simulink subsystem "button_filter"  (R2022b)
settings: Solver=VariableStepAuto  StartTime=0.0  StopTime=0.02  RelTol=1e-3
libraries: simulink x8
settings Model: DefaultTestHarness=button_filter_harness  Creator=andre  LastModifiedBy=andre
settings ModelReferenceCC: EnableRefExpFcnMdlSchedulingChecks=on

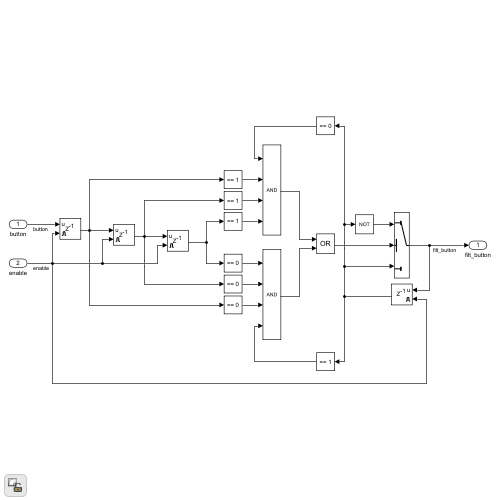
[thumbnail: Simulink's stored preview of the top-level diagram]
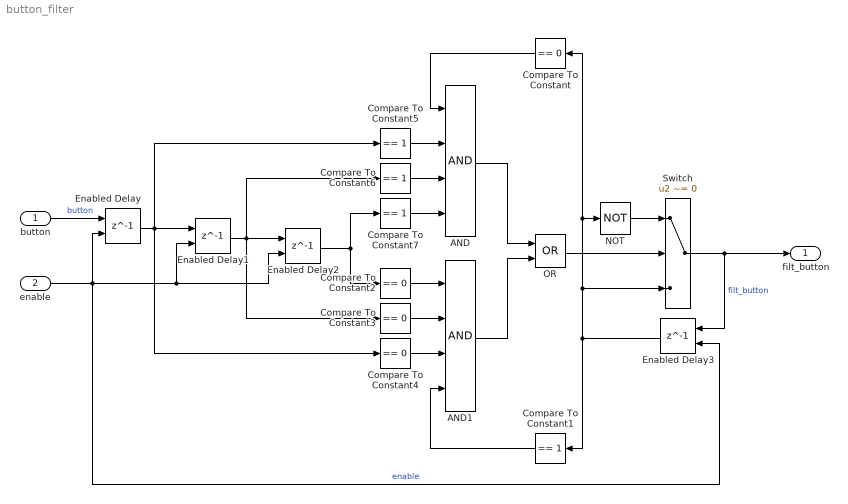
== system button_filter ==
  button : Inport  OutDataTypeStr=boolean  PortDimensions=1
  enable : Inport  Port=2  OutDataTypeStr=boolean  PortDimensions=1
  AND : Logic  Inputs=4  AllPortsSameDT=off  OutDataTypeStr=boolean
  AND1 : Logic  Inputs=4  AllPortsSameDT=off  OutDataTypeStr=boolean
  Compare To Constant{,2..4} (4 alike) : simulink/Logic and Bit Operations/Compare To Constant  relop===  const=0  OutDataTypeStr=boolean
  Compare To Constant{1,5..7} (4 alike) : simulink/Logic and Bit Operations/Compare To Constant  relop===  const=1  OutDataTypeStr=boolean
  Enabled Delay{,1..3} (4 alike) : Delay  DelayLength=1  ShowEnablePort=on
      settings: InputPortMap=u0,e6
  NOT : Logic  Operator=NOT  AllPortsSameDT=off  OutDataTypeStr=boolean
  OR : Logic  Operator=OR  AllPortsSameDT=off  OutDataTypeStr=boolean
  Switch : Switch  Criteria=u2 ~= 0  SaturateOnIntegerOverflow=off  InputSameDT=off
  filt_button : Outport  OutDataTypeStr=boolean  PortDimensions=1
  wires:
  button/1 -> Enabled Delay/1  "button"
  Switch/1 -> filt_button/1, Enabled Delay3/1  "filt_button"
  Compare To Constant3/1 -> AND1/2
  Compare To Constant1/1 -> AND1/4
  Enabled Delay2/1 -> Compare To Constant2/1, Compare To Constant7/1
  Enabled Delay3/1 -> Switch/3, NOT/1, Compare To Constant/1, Compare To Constant1/1
  AND1/1 -> OR/2
  Compare To Constant6/1 -> AND/3
  Compare To Constant7/1 -> AND/4
  OR/1 -> Switch/2
  Compare To Constant/1 -> AND/1
  AND/1 -> OR/1
  Enabled Delay/1 -> Compare To Constant5/1, Enabled Delay1/1, Compare To Constant4/1
  Compare To Constant4/1 -> AND1/3
  Compare To Constant2/1 -> AND1/1
  Compare To Constant5/1 -> AND/2
  NOT/1 -> Switch/1
  Enabled Delay1/1 -> Compare To Constant6/1, Compare To Constant3/1, Enabled Delay2/1
  enable/1 -> Enabled Delay1/2, Enabled Delay2/2, Enabled Delay/2, Enabled Delay3/2  "enable"
